simulink model "UnicycleWithSensor2019b_Solution"  (R2023b)
settings: Solver=VariableStepAuto  StartTime=0.0  StopTime=inf  RelTol=1e-3
values from neighbouring files (symbols this model uses):
  P = 10    [go2goalWithSensor.m]
  thetainit = 0    [go2goalWithSensor.m]
  tol = 0.1    [go2goalWithSensor.m]
  xg = gPos(2)    [go2goalWithSensor.m]
  xinit = sPos(2)    [go2goalWithSensor.m]
  yg = gPos(1)    [go2goalWithSensor.m]
  yinit = sPos(1)    [go2goalWithSensor.m]
  Z = ones(SizeX, SizeY)*255    [CreateMaze.m]
libraries: slpidlib x1, simulink_extras x1
settings Model: Creator=npn01  LastModifiedBy=jake9
settings SolverCC: AlgebraicLoopSolver=TrustRegion
settings DebuggingCC: UnconnectedInputMsg=warning  UnconnectedOutputMsg=warning  UnconnectedLineMsg=warning  UnderSpecifiedDimensionMsg=warning  ArithmeticOperatorsInVariantConditions=warning
settings ModelReferenceCC: EnableRefExpFcnMdlSchedulingChecks=on
settings SFSimCC: CustomCodeUndefinedFunction=UseInterfaceOnly

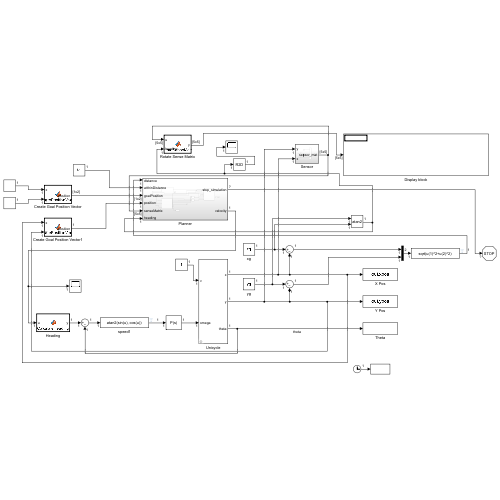
[thumbnail: Simulink's stored preview of the top-level diagram]
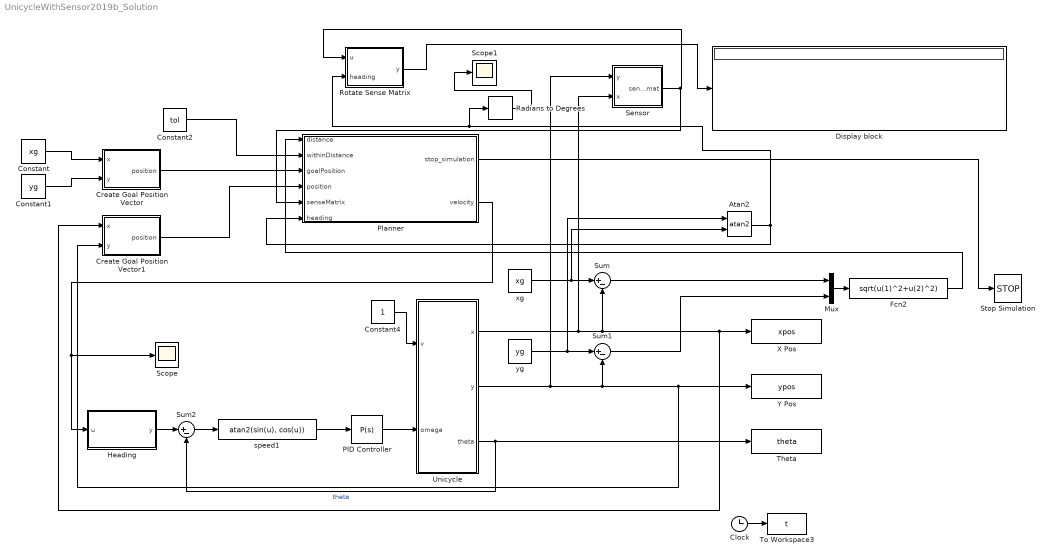
== system UnicycleWithSensor2019b_Solution ==
  Atan2 : Trigonometry  Operator=atan2
  Clock : Clock
  Constant : Constant  Value=xg
  Constant1 : Constant  Value=yg
  Constant2 : Constant  Value=tol
  Constant4 : Constant
  Create Goal Position Vector : MATLAB Function  TreatAsAtomicUnit=on
  Create Goal Position Vector1 : MATLAB Function  TreatAsAtomicUnit=on
  Display block : Display
  Fcn2 : Fcn  Expr=sqrt(u(1)^2+u(2)^2)
  Heading : MATLAB Function  TreatAsAtomicUnit=on
  Mux : Mux  Inputs=2
  PID Controller : slpidlib/PID Controller  Controller=P  Form=Parallel  TimeDomain=Continuous-time  UseExternalTs=off  SampleTime=-1  IntegratorMethod=Forward Euler  FilterMethod=Forward Euler  ControllerParametersSource=internal  P=P  I=0  UseKiTs=off  D=0  N=100  UseFilter=on  TunerSelectOption=Transfer Function Based (PID Tuner App)  InitialConditionSource=internal  InitialConditionForIntegrator=0  InitialConditionForFilter=0  DifferentiatorICPrevScaledInput=0  ExternalReset=none  TrackingMode=off  Kt=1  LimitOutput=off  SatLimitsSource=internal  UpperSaturationLimit=inf  LowerSaturationLimit=-inf  LinearizeAsGain=on  AntiWindupMode=none  Kb=1  LimitIntegrator=off  UpperIntegratorSaturationLimit=inf  LowerIntegratorSaturationLimit=-inf  POutMin=[]  POutMax=[]  IOutMin=[]  IOutMax=[]  DOutMin=[]  DOutMax=[]  NOutMin=[]  NOutMax=[]  SumOutMin=[]  SumOutMax=[]  SaturationOutMin=[]  SaturationOutMax=[]  PParamMin=[]  PParamMax=[]  IParamMin=[]  IParamMax=[]  DParamMin=[]  DParamMax=[]  NParamMin=[]  NParamMax=[]  KbParamMin=[]  KbParamMax=[]  KtParamMin=[]  KtParamMax=[]  KbOutMin=[]  KbOutMax=[]  KtOutMin=[]  KtOutMax=[]  IntegratorOutMin=[]  IntegratorOutMax=[]  FilterOutMin=[]  FilterOutMax=[]  SumI1OutMin=[]  SumI1OutMax=[]  SumI2OutMin=[]  SumI2OutMax=[]  SumI3OutMin=[]  SumI3OutMax=[]  SumI4OutMin=[]  SumI4OutMax=[]  SumDOutMin=[]  SumDOutMax=[]  DifferentiatorOutMin=[]  DifferentiatorOutMax=[]  FilterDiffOutCoefMin=[]  FilterDiffOutCoefMax=[]  ReciprocalOutMin=[]  ReciprocalOutMax=[]  SumDenOutMin=[]  SumDenOutMax=[]  SumNumOutMin=[]  SumNumOutMax=[]  DivideOutMin=[]  DivideOutMax=[]  UdiffTsProdOutMin=[]  UdiffTsProdOutMax=[]  NTsProdOutMin=[]  NTsProdOutMax=[]  UintegralTsProdOutMin=[]  UintegralTsProdOutMax=[]  UngainTsProdOutMin=[]  UngainTsProdOutMax=[]  ClampingZeroOutDataTypeStr=Inherit: Inherit via back propagation  ClampingZeroOutMin=[]  ClampingZeroOutMax=[]  FilterDenConstantOutDataTypeStr=Inherit: Inherit via back propagation  FilterDenConstantOutMin=[]  FilterDenConstantOutMax=[]  PCopyOutDataTypeStr=Inherit: Inherit via back propagation  PCopyOutMin=[]  PCopyOutMax=[]  NCopyOutDataTypeStr=Inherit: Inherit via back propagation  NCopyOutMin=[]  NCopyOutMax=[]  IntegratorContinuousStateAttributes=''  IntegratorStateMustResolveToSignalObject=off  IntegratorRTWStateStorageClass=Auto  FilterContinuousStateAttributes=''  FilterStateMustResolveToSignalObject=off  FilterRTWStateStorageClass=Auto  ParallelPVariant=InternalParameters  IdealPVariant=Disabled  IVariant=Disabled  DVariant=Disabled  IntegratorVariant=Disabled  SatVariant=Disabled  AWVariant=Disabled  PCopyVariant=Disabled  TRVariant=Disabled  FdbkBlocksVariant=Forward  IdealPFdbkVariant=Disabled  SatFdbkVariant=Disabled  DerivativeFilterVariant=Disabled  NVariant=Disabled  NCopyVariant=Disabled_SignalSpec  FilterICVariant=Disabled  IntegratorICVariant=Disabled  ExternalResetVariant=Disabled  TRSumVariant=Passthrough  SumFdbkVariant=Disabled  SumVariant=Passthrough_P  TsampFilterVariant=InternalTs  TsampNgainVariant=Passthrough  TsampIntegralVariant=Disabled_SignalSpec  ExternalSaturationOutDataTypeStr=Inherit: Same as second input
  Planner : Subsystem
  Radians to Degrees : simulink_extras/Transformations/Radians to Degrees
  Rotate Sense Matrix : MATLAB Function  TreatAsAtomicUnit=on
  Scope : Scope
  Scope1 : Scope
  Sensor : Subsystem
  Stop Simulation : Stop
  Sum : Sum  Inputs=|+-
  Sum1 : Sum  Inputs=|+-
  Sum2 : Sum  Inputs=|+-
  Theta : ToWorkspace  VariableName=theta  SampleTime=-1
  To Workspace3 : ToWorkspace  VariableName=t  SampleTime=-1
      settings: Save2DSignal=2-D array (concatenate along first dimension)
  Unicycle : Subsystem  mask{x0=xinit, y0=yinit, theta0=thetainit}
      mask DialogControl Control4 Prompt: Enter x initial position
      mask DialogControl Control2 Prompt: Enter y initial position
      mask DialogControl Control3 Prompt: Enter initial theta angle
      mask DialogControl Control6 Prompt: Any text you want
  X Pos : ToWorkspace  VariableName=xpos  SampleTime=-1
  Y Pos : ToWorkspace  VariableName=ypos  SampleTime=-1
  speed1 : Fcn  Expr=atan2(sin(u), cos(u))
  xg : Constant  Value=xg
  yg : Constant  Value=yg
  wires:
  xg/1 -> Atan2/2, Sum/1
  Unicycle/1(x) -> Sensor/2(x), Create Goal Position Vector1/1(x), X Pos/1, Sum/2
  yg/1 -> Atan2/1, Sum1/1
  Unicycle/2(y) -> Sensor/1(y), Sum1/2, Create Goal Position Vector1/2(y), Y Pos/1
  Sum/1 -> Mux/1
  Unicycle/3(theta) -> Theta/1, Sum2/2  "theta"
  PID Controller/1 -> Unicycle/2(omega)
  Sum2/1 -> speed1/1
  Clock/1 -> To Workspace3/1
  Mux/1 -> Fcn2/1
  Sum1/1 -> Mux/2
  Sensor/1(sensor_mat) -> Planner/5(senseMatrix), Rotate Sense Matrix/1(u)
  Constant/1 -> Create Goal Position Vector/1(x)
  Constant1/1 -> Create Goal Position Vector/2(y)
  speed1/1 -> PID Controller/1
  Heading/1(y) -> Sum2/1
  Planner/2(velocity) -> Scope/1, Heading/1(u)
  Fcn2/1 -> Planner/1(distance)
  Constant2/1 -> Planner/2(withinDistance)
  Planner/1(stop_simulation) -> Stop Simulation/1
  Constant4/1 -> Unicycle/1(v)
  Create Goal Position Vector/1(position) -> Planner/3(goalPosition)
  Create Goal Position Vector1/1(position) -> Planner/4(position)
  Rotate Sense Matrix/1(y) -> Display block/1
  Atan2/1 -> Radians to Degrees/1, Rotate Sense Matrix/2(heading), Planner/6(heading)
  Radians to Degrees/1 -> Scope1/1

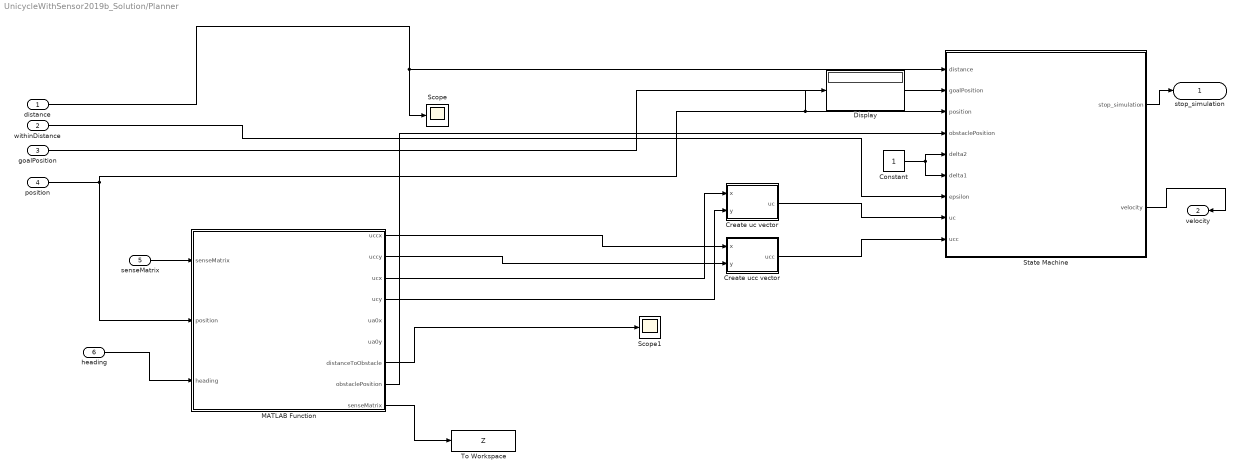
== system UnicycleWithSensor2019b_Solution/Planner ==
  distance : Inport
  withinDistance : Inport  Port=2
  goalPosition : Inport  Port=3
  position : Inport  Port=4
  senseMatrix : Inport  Port=5
  heading : Inport  Port=6
  Constant : Constant
  Create uc vector : MATLAB Function  TreatAsAtomicUnit=on
  Create ucc vector : MATLAB Function  TreatAsAtomicUnit=on
  Display : Display
  MATLAB Function : MATLAB Function  TreatAsAtomicUnit=on
  Scope : Scope
  Scope1 : Scope
  State Machine : Stateflow chart  TreatAsAtomicUnit=on
      settings: PortSchema="{\"entries\":[{\"content\":{\"sides\":[{\"content\":{\"connectorIds\":[\"In1\",\"In2\",\"In3\",\"In4\",\"In6\",\"In5\",\"In7\",\"In8\",\"In9\"]},\"type\":\"ConnectorPlacement.EquallySpacedRectSide\",\"uuid\":\"f7a5406f-d8ab-48f3-afc0-a6a97f8edc89\"},{\"content\":{\"connectorIds\":[\"Out1\",\"Out2\"],\"side\":\"RIGHT\"},\"type\":\"ConnectorPlacement.EquallySpacedRectSide\",\"uuid\":\"30b2deb1-2503-41d9-93ae-a7b3e9c8e922\"},{\"content\":{\"side\":\"TOP\"},\"type\":\"ConnectorPlacement.EquallySpacedRectSide\",\"uuid\":\"641fbf2e-2a84-40cd-8715-741285d67b9e\"}]},\"type\":\"ConnectorPlacement.EquallySpacedConnector\",\"uuid\":\"1a9f3f1e-ed88-4022-9191-699bf4a06c60\"}],\"packageUris\":[\"http://schema.mathworks.com/mf0/Connector/R2020b\"],\"version\":\"1.0\"}"
  To Workspace : ToWorkspace  VariableName=Z  SaveFormat=Timeseries  SampleTime=-1
  stop_simulation : Outport
  velocity : Outport  Port=2
  wires:
  distance/1 -> Scope/1, State Machine/1(distance)
  State Machine/2(velocity) -> velocity/1
  withinDistance/1 -> State Machine/7(epsilon)
  goalPosition/1 -> State Machine/2(goalPosition)
  State Machine/1(stop_simulation) -> stop_simulation/1
  position/1 -> MATLAB Function/2(position), Display/1, State Machine/3(position)
  senseMatrix/1 -> MATLAB Function/1("senseMatrix ")
  MATLAB Function/7(distanceToObstacle) -> Scope1/1
  MATLAB Function/9(senseMatrix) -> To Workspace/1
  MATLAB Function/1(uccx) -> Create ucc vector/1(x)
  MATLAB Function/2(uccy) -> Create ucc vector/2(y)
  heading/1 -> MATLAB Function/3(heading)
  MATLAB Function/3(ucx) -> Create uc vector/1(x)
  MATLAB Function/4(ucy) -> Create uc vector/2(y)
  MATLAB Function/8(obstaclePosition) -> State Machine/4(obstaclePosition)
  Constant/1 -> State Machine/5(delta1), State Machine/6(delta2)
  Create uc vector/1(uc) -> State Machine/8(uc)
  Create ucc vector/1(ucc) -> State Machine/9(ucc)

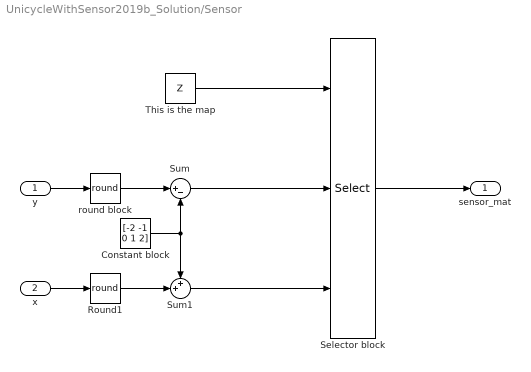
== system UnicycleWithSensor2019b_Solution/Sensor ==
  y : Inport
  x : Inport  Port=2
  Constant block : Constant  Value=[-2 -1 0 1 2]
  Round1 : Rounding  Operator=round
  Selector block : Selector  NumberOfDimensions=2  InputPortWidth=3  IndexOptions=Index vector (port),Index vector (port)  Indices=[1 3],1  OutputSizes=1,1
  Sum : Sum  Inputs=|+-  OutDataTypeStr=int32  RndMeth=Round
  Sum1 : Sum  Inputs=++|  OutDataTypeStr=int32  RndMeth=Round
  This is the map : Constant  Value=Z  VectorParams1D=off
  round block : Rounding  Operator=round
  sensor_mat : Outport
  wires:
  This is the map/1 -> Selector block/1
  Constant block/1 -> Sum1/1, Sum/2
  Sum/1 -> Selector block/2
  Sum1/1 -> Selector block/3
  Selector block/1 -> sensor_mat/1
  y/1 -> round block/1
  round block/1 -> Sum/1
  x/1 -> Round1/1
  Round1/1 -> Sum1/2

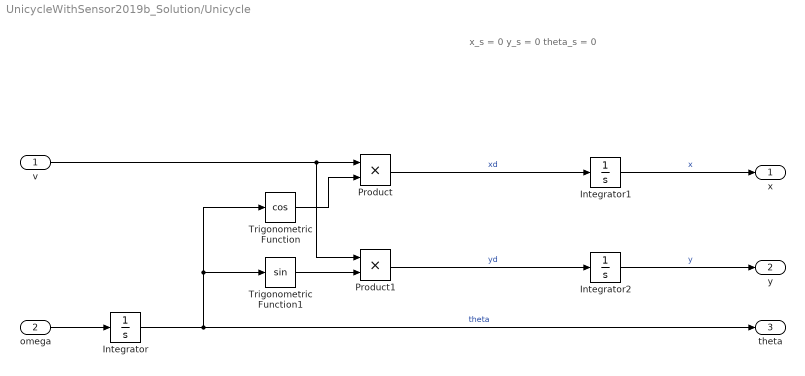
== system UnicycleWithSensor2019b_Solution/Unicycle ==
  note: x_s = 0
      | y_s = 0
      | theta_s = 0
  v : Inport
  omega : Inport  Port=2
  Integrator : Integrator  InitialCondition=theta0
  Integrator1 : Integrator  InitialCondition=x0
  Integrator2 : Integrator  InitialCondition=y0
  Product : Product
  Product1 : Product
  Trigonometric Function : Trigonometry  Operator=cos
  Trigonometric Function1 : Trigonometry
  x : Outport
  y : Outport  Port=2
  theta : Outport  Port=3
  wires:
  Product1/1 -> Integrator2/1  "yd"
  Integrator2/1 -> y/1  "y"
  v/1 -> Product1/1, Product/1
  Integrator/1 -> theta/1, Trigonometric Function1/1, Trigonometric Function/1  "theta"
  Product/1 -> Integrator1/1  "xd"
  omega/1 -> Integrator/1
  Trigonometric Function/1 -> Product/2
  Integrator1/1 -> x/1  "x"
  Trigonometric Function1/1 -> Product1/2

== stateflow chart UnicycleWithSensor2019b_Solution/Planner/State Machine ==
  state stop
    entry:
    stop_simulation=true;
  state gtg_state
    entry:
    obstacleToPositionDistance = 0;
    during:
    velocity = goalPosition - position;
    obstacleToPosition = obstaclePosition - position;
    obstacleToPositionDistance = sqrt(obstacleToPosition(1)^2 + obstacleToPosition(2)^2);
    product_gtg_ucc = sum((goalPosition - position) .* ucc);
    product_gtg_uc = sum((goalPosition - position) .* uc);
  state uc_state
    entry:
    positionToGoal = goalPosition - position;
    d = sqrt(positionToGoal(1)^2 + positionToGoal(2)^2);
    during:
    velocity = uc;
    positionToGoal = goalPosition - position;
  state ucc_state
    entry:
    positionToGoal = goalPosition - position;
    d = sqrt(positionToGoal(1)^2 + positionToGoal(2)^2);
    during:
    velocity = ucc;
    positionToGoal = goalPosition - position;
    product_ao_gtg = sum(obstacleToPosition .* (goalPosition - position));
  state ua0_state
    during:
    velocity = obstaclePosition - position;
    obstacleToPosition = obstaclePosition - position;
    obstacleToPositionDistance = sqrt(obstacleToPosition(1)^2 + obstacleToPosition(2)^2);
    product_gtg_ucc = sum((goalPosition - position) .* ucc);
    product_gtg_uc = sum((goalPosition - position) .* uc);
  gtg_state -> stop [order 1] : [distance <= epsilon]
  (default) -> gtg_state
  gtg_state -> uc_state [order 3] : [obstacleToPositionDistance < delta1 && product_gtg_uc > 0]
  gtg_state -> ucc_state [order 2] : [obstacleToPositionDistance < delta1 && product_gtg_ucc > 0]
  ucc_state -> gtg_state [order 2] : [positionToGoal < d && product_ao_gtg > 0]
  uc_state -> gtg_state [order 2] : [positionToGoal < d && product_ao_gtg > 0]
  ua0_state -> uc_state [order 2] : [obstacleToPositionDistance >= delta2 && product_gtg_uc > 0]
  uc_state -> ua0_state [order 1] : [obstacleToPositionDistance < delta2]
  ucc_state -> ua0_state [order 1] : [obstacleToPositionDistance < delta2]
  ua0_state -> ucc_state [order 1] : [obstacleToPositionDistance >= delta2 && product_gtg_ucc > 0]
  data: distance input; stop_simulation output; velocity output; goalPosition input; position input; obstaclePosition input; delta1 input; delta2 input; epsilon input; uc input; ucc input; product_gtg_ucc local =0; product_gtg_uc local =0; obstacleToPosition local; obstacleToPositionDistance local =0; positionToGoal local; d local =0; product_ao_gtg local =0

== matlab function UnicycleWithSensor2019b_Solution/Heading ==
  data: u input; y output
function y = CalculateHeading(u)

y = atan2(u(2), u(1));

== matlab function UnicycleWithSensor2019b_Solution/Planner/MATLAB Function ==
  data: senseMatrix input; uccx output; uccy output; position input; ucx output; ucy output; ua0x output; ua0y output; distanceToObstacle output; obstaclePosition output; senseMatrix output; heading input
function [uccx, uccy, ucx, ucy, ua0x, ua0y, distanceToObstacle, obstaclePosition, senseMatrix] = CalculateObstacleDirectionsAndPosition(senseMatrix, position, heading)

thetaC = pi/2;
thetaCC = -pi/2;
ucRotation = [cos(thetaC), -sin(thetaC);
              sin(thetaC), cos(thetaC)]';

uccRotation = [cos(thetaCC), -sin(thetaCC);
               sin(thetaCC), cos(thetaCC)]';

rotation = [cos(heading), -sin(heading);
            sin(heading), cos(heading)]';

uc = [0 0];
ucc = [0 0];
distanceToObstacle = 100;
obstaclePosition = [0 0];
ua0x = 0;
ua0y = 0;
uccx = 0;
uccy = 0;
ucx = 0;
ucy = 0;

xGlobal = rotation * [1; 0] - position';
mag = sqrt(xGlobal(1)^2 + xGlobal(2)^2);
xGlobal = xGlobal ./ mag;

value = senseMatrix(3 + round(xGlobal(1)), 3 + round(xGlobal(2)));

% Obstacle in front of the robot.
if value == 0
    distanceToObstacle = 1;
    uc = (ucRotation * [-1; 0]).';
    ucc = (uccRotation * [-1; 0]).';
    uccx = ucc(1);
    uccy = ucc(2);
    ucx = uc(1);
    ucy = uc(2);
    ua0x = 0;
    ua0y = -1;
    obstaclePosition = [3 + round(xGlobal(1)), 3 + round(xGlobal(2))];
end

== matlab function UnicycleWithSensor2019b_Solution/Rotate Sense Matrix ==
  data: u input; y output; heading input
function y = RotateSenseMatrix(u, heading)

y = rot90(u, -round((((pi/2) - heading) / (pi/2))));
end

== matlab function UnicycleWithSensor2019b_Solution/Planner/Create ucc vector ==
  data: x input; ucc output; y input
function ucc = CreatePositionVector(x, y)

ucc = [x y];
end

== matlab function UnicycleWithSensor2019b_Solution/Planner/Create uc vector ==
  data: x input; uc output; y input
function uc = CreatePositionVector(x, y)

uc = [x y];
end

== matlab function UnicycleWithSensor2019b_Solution/Create Goal Position Vector1 ==
  data: x input; position output; y input
function position = CreatePositionVector(x, y)

position = [x y];
end

== matlab function UnicycleWithSensor2019b_Solution/Create Goal Position Vector ==
  data: x input; position output; y input
function position = CreatePositionVector(x, y)

position = [x y];
end
